simulink model "SIL_HarnessTest"  (R2020a)
settings: Solver=FixedStepDiscrete  StartTime=0.0  StopTime=10.0  FixedStep=1  RelTol=1e-3
settings Model: Creator=ashok  LastModifiedBy=ashok
settings DataIOCC: LoadExternalInput=on  InspectSignalLogs=on  ReturnWorkspaceOutputs=off  OutputSaveName=mdl_out  LoggingToFile=on  LoggingFileName=mdl_out.mat
settings OptimizationCC: DefaultParameterBehavior=Inlined  EnhancedBackFolding=on  PassReuseOutputArgsAs=Individual arguments  ZeroExternalMemoryAtStartup=off  ZeroInternalMemoryAtStartup=off  OptimizeBlockOrder=speed  DifferentSizesBufferReuse=on  OptimizationCustomize=off  EfficientTunableParamExpr=on
settings DebuggingCC: ParameterTunabilityLossMsg=error
settings HardwareCC: ProdBitPerPointer=32  ProdBitPerSizeT=32  ProdBitPerPtrDiffT=32  ProdLargestAtomicFloat=None  ProdWordSize=32  ProdHWDeviceType=Atmel->AVR (32-bit)
settings SFSimCC: MATLABDynamicMemAlloc=off
settings RTWCC: SystemTargetFile=ert.tlc  TemplateMakefile=ert_default_tmf  PortableWordSizes=on
settings CodeAppCC: ForceParamTrailComments=on  IgnoreCustomStorageClasses=off  OperatorAnnotations=on  SimulinkDataObjDesc=on  SFDataObjDesc=on  InsertBlockDesc=on
settings ERTTargetCC: TargetLangStandard=C99 (ISO)  GenerateSampleERTMain=on  InlinedParameterPlacement=NonHierarchical  ERTCustomFileTemplate=example_file_process.tlc

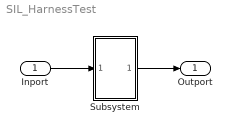
== system SIL_HarnessTest ==
  Inport : Inport
  Subsystem : Subsystem  TreatAsAtomicUnit=on
  Outport : Outport
  wires:
  Inport/1 -> Subsystem/1(In1)
  Subsystem/1(Out1) -> Outport/1

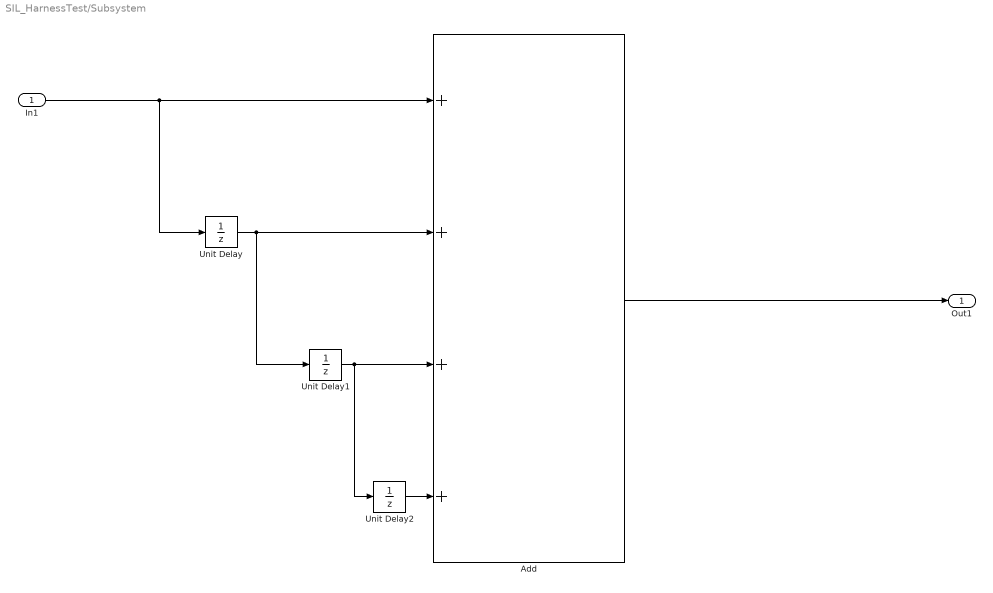
== system SIL_HarnessTest/Subsystem ==
  In1 : Inport
  Add : Sum  Inputs=++++
  Unit Delay : UnitDelay  SampleTime=-1  HasFrameUpgradeWarning=on
  Unit Delay1 : UnitDelay  SampleTime=-1  HasFrameUpgradeWarning=on
  Unit Delay2 : UnitDelay  SampleTime=-1  HasFrameUpgradeWarning=on
  Out1 : Outport
  wires:
  Unit Delay1/1 -> Unit Delay2/1, Add/3
  Add/1 -> Out1/1
  Unit Delay/1 -> Unit Delay1/1, Add/2
  In1/1 -> Unit Delay/1, Add/1
  Unit Delay2/1 -> Add/4
